simulink model "greenScience"  (R2023b)
settings: Solver=VariableStepAuto  StartTime=0.0  StopTime=16  RelTol=1e-3
settings Model: Creator=Brenton  LastModifiedBy=Brenton

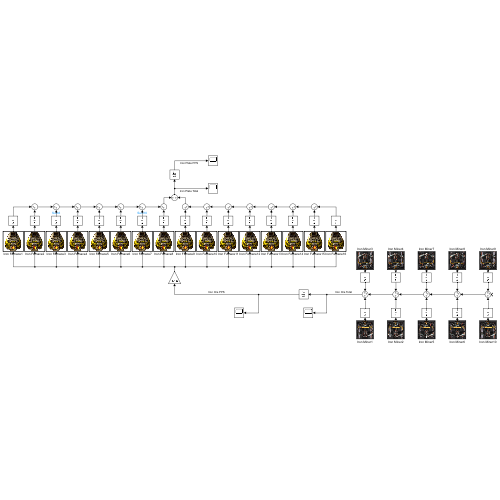
[thumbnail: Simulink's stored preview of the top-level diagram]
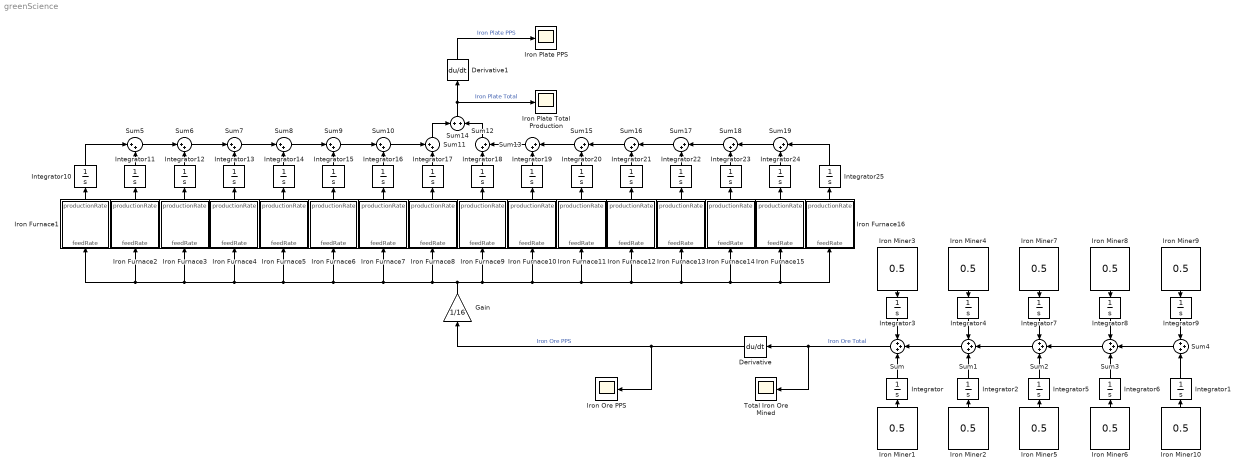
== system greenScience ==
  Derivative : Derivative
  Derivative1 : Derivative
  Gain : Gain  Gain=1/16
  Integrator{,1..25} (26 alike) : Integrator
  Iron Furnace1 : MATLAB Function  TreatAsAtomicUnit=on
  Iron Furnace10 : MATLAB Function  TreatAsAtomicUnit=on
  Iron Furnace11 : MATLAB Function  TreatAsAtomicUnit=on
  Iron Furnace12 : MATLAB Function  TreatAsAtomicUnit=on
  Iron Furnace13 : MATLAB Function  TreatAsAtomicUnit=on
  Iron Furnace14 : MATLAB Function  TreatAsAtomicUnit=on
  Iron Furnace15 : MATLAB Function  TreatAsAtomicUnit=on
  Iron Furnace16 : MATLAB Function  TreatAsAtomicUnit=on
  Iron Furnace2 : MATLAB Function  TreatAsAtomicUnit=on
  Iron Furnace3 : MATLAB Function  TreatAsAtomicUnit=on
  Iron Furnace4 : MATLAB Function  TreatAsAtomicUnit=on
  Iron Furnace5 : MATLAB Function  TreatAsAtomicUnit=on
  Iron Furnace6 : MATLAB Function  TreatAsAtomicUnit=on
  Iron Furnace7 : MATLAB Function  TreatAsAtomicUnit=on
  Iron Furnace8 : MATLAB Function  TreatAsAtomicUnit=on
  Iron Furnace9 : MATLAB Function  TreatAsAtomicUnit=on
  Iron Miner{1..10} (10 alike) : Constant  Value=0.5
      Iron Miner1 mask Display: image('electricMiningDrill_up.png');
      Iron Miner10 mask Display: image('electricMiningDrill_up.png');
      Iron Miner2 mask Display: image('electricMiningDrill_up.png');
      Iron Miner3 mask Display: image('electricMiningDrill_down.png');
      Iron Miner4 mask Display: image('electricMiningDrill_down.png');
      Iron Miner5 mask Display: image('electricMiningDrill_up.png');
      Iron Miner6 mask Display: image('electricMiningDrill_up.png');
      Iron Miner7 mask Display: image('electricMiningDrill_down.png');
      Iron Miner8 mask Display: image('electricMiningDrill_down.png');
      Iron Miner9 mask Display: image('electricMiningDrill_down.png');
  Iron Ore PPS : Scope
  Iron Plate PPS : Scope
  Iron Plate Total Production : Scope
  Sum{,1..4} (5 alike) : Sum  Inputs=+++
  Sum{5..10,12..13,15..19} (13 alike) : Sum  Inputs=|++
  Sum11 : Sum  Inputs=++|
  Sum14 : Sum  Inputs=+|+
  Total Iron Ore Mined : Scope
  wires:
  Iron Miner1/1 -> Integrator/1
  Sum/1 -> Derivative/1, Total Iron Ore Mined/1  "Iron Ore Total"
  Iron Miner2/1 -> Integrator2/1
  Integrator/1 -> Sum/3
  Integrator2/1 -> Sum1/3
  Iron Miner3/1 -> Integrator3/1
  Integrator3/1 -> Sum/1
  Iron Miner4/1 -> Integrator4/1
  Integrator4/1 -> Sum1/1
  Sum1/1 -> Sum/2
  Iron Miner8/1 -> Integrator8/1
  Integrator8/1 -> Sum3/1
  Integrator5/1 -> Sum2/3
  Integrator6/1 -> Sum3/3
  Iron Miner6/1 -> Integrator6/1
  Integrator7/1 -> Sum2/1
  Sum3/1 -> Sum2/2
  Iron Miner5/1 -> Integrator5/1
  Iron Miner7/1 -> Integrator7/1
  Sum2/1 -> Sum1/2
  Iron Miner9/1 -> Integrator9/1
  Integrator9/1 -> Sum4/1
  Iron Miner10/1 -> Integrator1/1
  Sum4/1 -> Sum3/2
  Integrator1/1 -> Sum4/3
  Derivative/1 -> Gain/1, Iron Ore PPS/1  "Iron Ore PPS"
  Gain/1 -> Iron Furnace10/1(feedRate), Iron Furnace14/1(feedRate), Iron Furnace16/1(feedRate), Iron Furnace15/1(feedRate), Iron Furnace13/1(feedRate), Iron Furnace12/1(feedRate), Iron Furnace11/1(feedRate), Iron Furnace9/1(feedRate), Iron Furnace8/1(feedRate), Iron Furnace7/1(feedRate), Iron Furnace6/1(feedRate), Iron Furnace5/1(feedRate), Iron Furnace3/1(feedRate), Iron Furnace2/1(feedRate), Iron Furnace1/1(feedRate), Iron Furnace4/1(feedRate)
  Iron Furnace1/1(productionRate) -> Integrator10/1
  Iron Furnace2/1(productionRate) -> Integrator11/1
  Iron Furnace4/1(productionRate) -> Integrator13/1
  Iron Furnace3/1(productionRate) -> Integrator12/1
  Iron Furnace8/1(productionRate) -> Integrator17/1
  Iron Furnace7/1(productionRate) -> Integrator16/1
  Iron Furnace6/1(productionRate) -> Integrator15/1
  Iron Furnace5/1(productionRate) -> Integrator14/1
  Iron Furnace12/1(productionRate) -> Integrator21/1
  Iron Furnace11/1(productionRate) -> Integrator20/1
  Iron Furnace16/1(productionRate) -> Integrator25/1
  Iron Furnace15/1(productionRate) -> Integrator24/1
  Iron Furnace10/1(productionRate) -> Integrator19/1
  Iron Furnace13/1(productionRate) -> Integrator22/1
  Iron Furnace14/1(productionRate) -> Integrator23/1
  Iron Furnace9/1(productionRate) -> Integrator18/1
  Integrator11/1 -> Sum5/2
  Integrator12/1 -> Sum6/2
  Integrator13/1 -> Sum7/2
  Integrator14/1 -> Sum8/2
  Integrator15/1 -> Sum9/2
  Integrator16/1 -> Sum10/2
  Sum9/1 -> Sum10/1
  Sum8/1 -> Sum9/1
  Sum7/1 -> Sum8/1
  Sum6/1 -> Sum7/1
  Sum5/1 -> Sum6/1
  Integrator10/1 -> Sum5/1
  Integrator17/1 -> Sum11/2
  Sum10/1 -> Sum11/1
  Integrator18/1 -> Sum12/1
  Sum11/1 -> Sum14/1
  Sum12/1 -> Sum14/2
  Integrator25/1 -> Sum19/1
  Integrator24/1 -> Sum19/2
  Sum19/1 -> Sum18/1
  Integrator23/1 -> Sum18/2
  Sum18/1 -> Sum17/1
  Integrator22/1 -> Sum17/2
  Sum17/1 -> Sum16/1
  Integrator21/1 -> Sum16/2
  Sum16/1 -> Sum15/1
  Integrator20/1 -> Sum15/2
  Sum15/1 -> Sum13/1
  Integrator19/1 -> Sum13/2
  Sum13/1 -> Sum12/2
  Sum14/1 -> Derivative1/1, Iron Plate Total Production/1  "Iron Plate Total"
  Derivative1/1 -> Iron Plate PPS/1  "Iron Plate PPS"

== matlab function greenScience/Iron Furnace16 ==
  data: feedRate input; productionRate output
function productionRate = fcn(feedRate)
    maxProductionRate = 0.3125; % per second
    materialRatioIO = 1;
    maxConsumptionRate = maxProductionRate * materialRatioIO;
    if feedRate * materialRatioIO >= maxConsumptionRate
        productionRate = maxProductionRate;
    else
        productionRate = feedRate;
    end
end

== matlab function greenScience/Iron Furnace9 ==
  data: feedRate input; productionRate output
function productionRate = fcn(feedRate)
    maxProductionRate = 0.3125; % per second
    materialRatioIO = 1;
    maxConsumptionRate = maxProductionRate * materialRatioIO;
    if feedRate * materialRatioIO >= maxConsumptionRate
        productionRate = maxProductionRate;
    else
        productionRate = feedRate;
    end
end

== matlab function greenScience/Iron Furnace1 ==
  data: feedRate input; productionRate output
function productionRate = fcn(feedRate)
    maxProductionRate = 0.3125; % per second
    materialRatioIO = 1;
    maxConsumptionRate = maxProductionRate * materialRatioIO;
    if feedRate * materialRatioIO >= maxConsumptionRate
        productionRate = maxProductionRate;
    else
        productionRate = feedRate;
    end
end

== matlab function greenScience/Iron Furnace3 ==
  data: feedRate input; productionRate output
function productionRate = fcn(feedRate)
    maxProductionRate = 0.3125; % per second
    materialRatioIO = 1;
    maxConsumptionRate = maxProductionRate * materialRatioIO;
    if feedRate * materialRatioIO >= maxConsumptionRate
        productionRate = maxProductionRate;
    else
        productionRate = feedRate;
    end
end

== matlab function greenScience/Iron Furnace4 ==
  data: feedRate input; productionRate output
function productionRate = fcn(feedRate)
    maxProductionRate = 0.3125; % per second
    materialRatioIO = 1;
    maxConsumptionRate = maxProductionRate * materialRatioIO;
    if feedRate * materialRatioIO >= maxConsumptionRate
        productionRate = maxProductionRate;
    else
        productionRate = feedRate;
    end
end

== matlab function greenScience/Iron Furnace5 ==
  data: feedRate input; productionRate output
function productionRate = fcn(feedRate)
    maxProductionRate = 0.3125; % per second
    materialRatioIO = 1;
    maxConsumptionRate = maxProductionRate * materialRatioIO;
    if feedRate * materialRatioIO >= maxConsumptionRate
        productionRate = maxProductionRate;
    else
        productionRate = feedRate;
    end
end

== matlab function greenScience/Iron Furnace6 ==
  data: feedRate input; productionRate output
function productionRate = fcn(feedRate)
    maxProductionRate = 0.3125; % per second
    materialRatioIO = 1;
    maxConsumptionRate = maxProductionRate * materialRatioIO;
    if feedRate * materialRatioIO >= maxConsumptionRate
        productionRate = maxProductionRate;
    else
        productionRate = feedRate;
    end
end

== matlab function greenScience/Iron Furnace7 ==
  data: feedRate input; productionRate output
function productionRate = fcn(feedRate)
    maxProductionRate = 0.3125; % per second
    materialRatioIO = 1;
    maxConsumptionRate = maxProductionRate * materialRatioIO;
    if feedRate * materialRatioIO >= maxConsumptionRate
        productionRate = maxProductionRate;
    else
        productionRate = feedRate;
    end
end

== matlab function greenScience/Iron Furnace8 ==
  data: feedRate input; productionRate output
function productionRate = fcn(feedRate)
    maxProductionRate = 0.3125; % per second
    materialRatioIO = 1;
    maxConsumptionRate = maxProductionRate * materialRatioIO;
    if feedRate * materialRatioIO >= maxConsumptionRate
        productionRate = maxProductionRate;
    else
        productionRate = feedRate;
    end
end

== matlab function greenScience/Iron Furnace10 ==
  data: feedRate input; productionRate output
function productionRate = fcn(feedRate)
    maxProductionRate = 0.3125; % per second
    materialRatioIO = 1;
    maxConsumptionRate = maxProductionRate * materialRatioIO;
    if feedRate * materialRatioIO >= maxConsumptionRate
        productionRate = maxProductionRate;
    else
        productionRate = feedRate;
    end
end

== matlab function greenScience/Iron Furnace2 ==
  data: feedRate input; productionRate output
function productionRate = fcn(feedRate)
    maxProductionRate = 0.3125; % per second
    materialRatioIO = 1;
    maxConsumptionRate = maxProductionRate * materialRatioIO;
    if feedRate * materialRatioIO >= maxConsumptionRate
        productionRate = maxProductionRate;
    else
        productionRate = feedRate;
    end
end

== matlab function greenScience/Iron Furnace11 ==
  data: feedRate input; productionRate output
function productionRate = fcn(feedRate)
    maxProductionRate = 0.3125; % per second
    materialRatioIO = 1;
    maxConsumptionRate = maxProductionRate * materialRatioIO;
    if feedRate * materialRatioIO >= maxConsumptionRate
        productionRate = maxProductionRate;
    else
        productionRate = feedRate;
    end
end

== matlab function greenScience/Iron Furnace12 ==
  data: feedRate input; productionRate output
function productionRate = fcn(feedRate)
    maxProductionRate = 0.3125; % per second
    materialRatioIO = 1;
    maxConsumptionRate = maxProductionRate * materialRatioIO;
    if feedRate * materialRatioIO >= maxConsumptionRate
        productionRate = maxProductionRate;
    else
        productionRate = feedRate;
    end
end

== matlab function greenScience/Iron Furnace13 ==
  data: feedRate input; productionRate output
function productionRate = fcn(feedRate)
    maxProductionRate = 0.3125; % per second
    materialRatioIO = 1;
    maxConsumptionRate = maxProductionRate * materialRatioIO;
    if feedRate * materialRatioIO >= maxConsumptionRate
        productionRate = maxProductionRate;
    else
        productionRate = feedRate;
    end
end

== matlab function greenScience/Iron Furnace14 ==
  data: feedRate input; productionRate output
function productionRate = fcn(feedRate)
    maxProductionRate = 0.3125; % per second
    materialRatioIO = 1;
    maxConsumptionRate = maxProductionRate * materialRatioIO;
    if feedRate * materialRatioIO >= maxConsumptionRate
        productionRate = maxProductionRate;
    else
        productionRate = feedRate;
    end
end

== matlab function greenScience/Iron Furnace15 ==
  data: feedRate input; productionRate output
function productionRate = fcn(feedRate)
    maxProductionRate = 0.3125; % per second
    materialRatioIO = 1;
    maxConsumptionRate = maxProductionRate * materialRatioIO;
    if feedRate * materialRatioIO >= maxConsumptionRate
        productionRate = maxProductionRate;
    else
        productionRate = feedRate;
    end
end
